simulink model "joystickRead"  (R2024a)
settings: configuration reference "standardSILConfiguraitonParams" (kept outside this file)
libraries: simulink x6
settings Model: Creator=jerem  LastModifiedBy=jerem
settings ConfigSetRef: SourceName=standardSILConfiguraitonParams  SourceLocation=Base Workspace

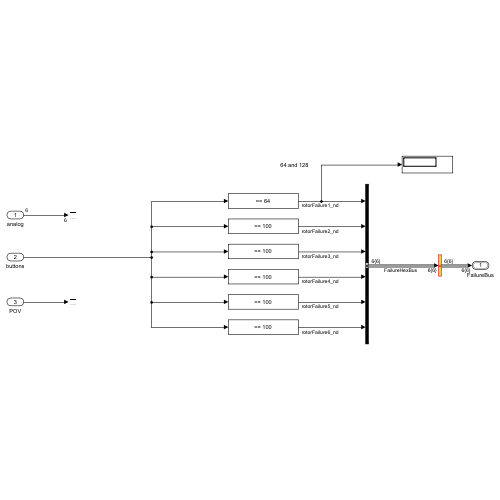
[thumbnail: Simulink's stored preview of the top-level diagram]
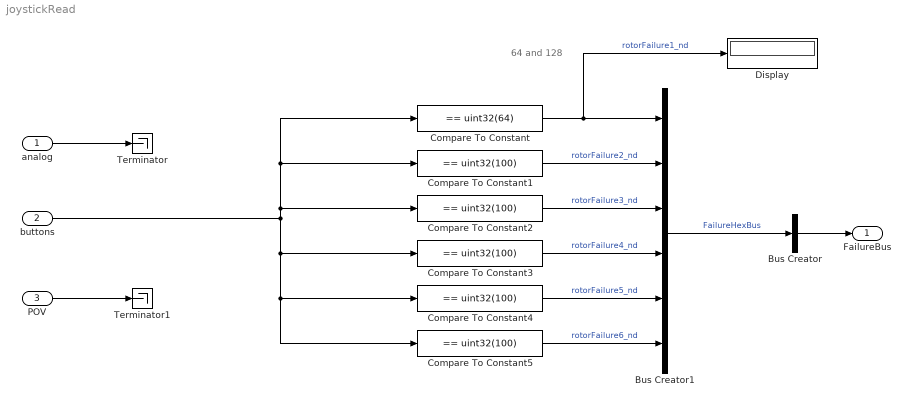
== system joystickRead ==
  note: 64 and 128
  analog : Inport  PortDimensions=6
  buttons : Inport  Port=2  OutDataTypeStr=uint32
  POV : Inport  Port=3
  Bus Creator : BusCreator  Inputs=1  OutDataTypeStr=Bus: FailureBus
  Bus Creator1 : BusCreator  Inputs=6  OutDataTypeStr=Bus: FailureHexBus
  Compare To Constant : simulink/Logic and Bit Operations/Compare To Constant  relop===  const=uint32(64)  OutDataTypeStr=boolean
  Compare To Constant{1..5} (5 alike) : simulink/Logic and Bit Operations/Compare To Constant  relop===  const=uint32(100)  OutDataTypeStr=boolean
  Display : Display
  Terminator : Terminator
  Terminator1 : Terminator
  FailureBus : Outport  OutDataTypeStr=Bus: FailureBus
  wires:
  analog/1 -> Terminator/1
  POV/1 -> Terminator1/1
  buttons/1 -> Compare To Constant/1, Compare To Constant1/1, Compare To Constant2/1, Compare To Constant3/1, Compare To Constant4/1, Compare To Constant5/1
  Bus Creator1/1 -> Bus Creator/1  "FailureHexBus"
  Bus Creator/1 -> FailureBus/1
  Compare To Constant/1 -> Display/1, Bus Creator1/1  "rotorFailure1_nd"
  Compare To Constant1/1 -> Bus Creator1/2  "rotorFailure2_nd"
  Compare To Constant2/1 -> Bus Creator1/3  "rotorFailure3_nd"
  Compare To Constant3/1 -> Bus Creator1/4  "rotorFailure4_nd"
  Compare To Constant4/1 -> Bus Creator1/5  "rotorFailure5_nd"
  Compare To Constant5/1 -> Bus Creator1/6  "rotorFailure6_nd"
